simulink model "CruiseControlSim"  (R2024a)
settings: Solver=ode45  StartTime=0.0  StopTime=Tf  RelTol=1e-4
values from neighbouring files (symbols this model uses):
  b0 = -336.4    [CruiseControlPlots.m]
  b1 = 23.2    [CruiseControlPlots.m]
  Fgrav = 1400    [CruiseControlPlots.m]
  Froll = 228    [CruiseControlPlots.m]
  k = 40    [CruiseControlPlots.m]
  m = 2085    [CruiseControlPlots.m]
  ubar = (b1 * 29 + (Froll + b0)) / k    (= 14.11)    [CruiseControlPlots.m]
  v0 = 29    [CruiseControlPlots.m]
settings Model: Creator=pjseiler  LastModifiedBy=xinchen
settings SolverCC: AlgebraicLoopSolver=TrustRegion
settings DebuggingCC: UnconnectedInputMsg=warning  UnconnectedOutputMsg=warning  UnconnectedLineMsg=warning
settings ModelReferenceCC: EnableRefExpFcnMdlSchedulingChecks=on
settings RTWCC: GPUComputeCapability=3.5  DLArmComputeVersion=19.05

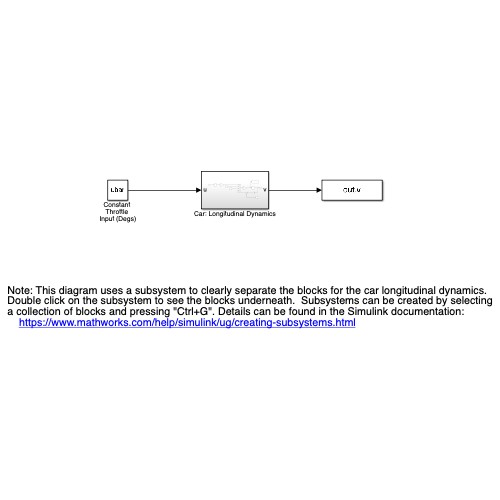
[thumbnail: Simulink's stored preview of the top-level diagram]
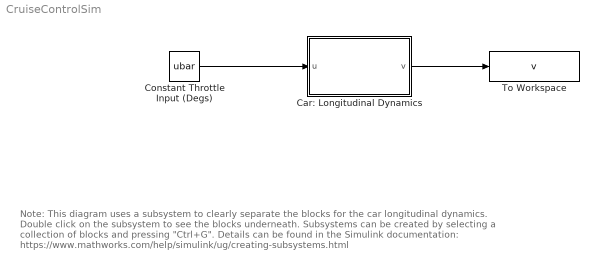
== system CruiseControlSim ==
  note: Note: This diagram uses a subsystem to clearly separate the blocks for the car longitudinal dynamics.
      | Double click on the subsystem to see the blocks underneath. Subsystems can be created by selecting
      | a collection of blocks and pressing "Ctrl+G". Details can be found in the Simulink documentation:
      | https://www.mathworks.com/help/simulink/ug/creating-subsystems.html
  Car: Longitudinal Dynamics : Subsystem
  Constant Throttle Input (Degs) : Constant  Value=ubar
  To Workspace : ToWorkspace  VariableName=v  SampleTime=-1
  wires:
  Car: Longitudinal Dynamics/1(v) -> To Workspace/1
  Constant Throttle Input (Degs)/1 -> Car: Longitudinal Dynamics/1(u)

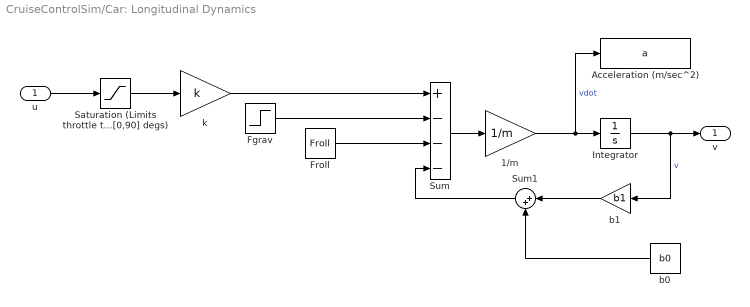
== system CruiseControlSim/Car: Longitudinal Dynamics ==
  u : Inport
  1/m : Gain  Gain=1/m
  Acceleration (m/sec^2) : ToWorkspace  VariableName=a  SampleTime=-1
  Fgrav : Step  Time=10  After=Fgrav  SampleTime=0
  Froll : Constant  Value=Froll
  Integrator : Integrator  InitialCondition=v0
  Saturation (Limits throttle to [0,90] degs) : Saturate  UpperLimit=90  LowerLimit=0
  Sum : Sum  Inputs=+---
  Sum1 : Sum  Inputs=|++
  b0 : Constant  Value=b0
  b1 : Gain  Gain=b1
  k : Gain  Gain=k
  v : Outport
  wires:
  Sum1/1 -> Sum/4
  Froll/1 -> Sum/3
  Fgrav/1 -> Sum/2
  k/1 -> Sum/1
  b0/1 -> Sum1/2
  b1/1 -> Sum1/1
  u/1 -> Saturation (Limits throttle to [0,90] degs)/1
  Sum/1 -> 1/m/1
  Integrator/1 -> v/1, b1/1  "v"
  1/m/1 -> Acceleration (m/sec^2)/1, Integrator/1  "vdot"
  Saturation (Limits throttle to [0,90] degs)/1 -> k/1
